simulink model "intento2"  (R2017b)
settings: Solver=VariableStepAuto  StartTime=0.0  StopTime=10.0  RelTol=1e-3
values from neighbouring files (symbols this model uses):
  kd = eval(S.kd)    [Lab4.m]    (also in Lab4Final.m; Lab4intento2.m; Lab4intento3.m)
  ki = eval(S.ki)    [Lab4.m]    (also in Lab4Final.m; Lab4intento2.m; Lab4intento3.m)
  ki2 = eval(S.ki2)    [Lab4Final.m]    (also in Lab4intento2.m)
  ki3 = eval(S.ki3)    [Lab4intento2.m]
  kp = eval(S.kp)    [Lab4.m]    (also in Lab4Final.m; Lab4intento2.m; Lab4intento3.m)
settings Model: Creator=Cx001la  LastModifiedBy=Cx001la

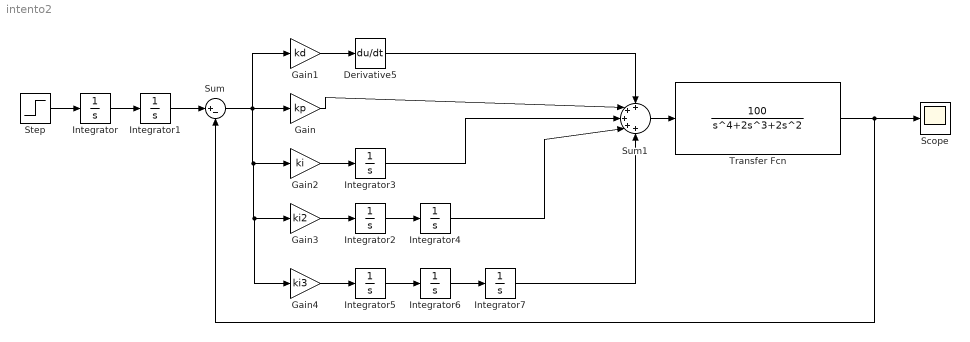
== system intento2 ==
  Derivative5 : Derivative
  Gain : Gain  Gain=kp
  Gain1 : Gain  Gain=kd
  Gain2 : Gain  Gain=ki
  Gain3 : Gain  Gain=ki2
  Gain4 : Gain  Gain=ki3
  Integrator{,1..7} (8 alike) : Integrator
  Scope : Scope
  Step : Step  Time=0  SampleTime=0
  Sum : Sum  Inputs=|+-
  Sum1 : Sum  Inputs=+++++
  Transfer Fcn : TransferFcn  Numerator=[100]  Denominator=[1 2 2 0 0]
  wires:
  Transfer Fcn/1 -> Scope/1, Sum/2
  Sum1/1 -> Transfer Fcn/1
  Integrator1/1 -> Sum/1
  Step/1 -> Integrator/1
  Sum/1 -> Gain1/1, Gain4/1, Gain3/1, Gain2/1, Gain/1
  Integrator/1 -> Integrator1/1
  Gain/1 -> Sum1/2
  Gain1/1 -> Derivative5/1
  Derivative5/1 -> Sum1/1
  Gain2/1 -> Integrator3/1
  Gain3/1 -> Integrator2/1
  Integrator2/1 -> Integrator4/1
  Gain4/1 -> Integrator5/1
  Integrator5/1 -> Integrator6/1
  Integrator6/1 -> Integrator7/1
  Integrator7/1 -> Sum1/5
  Integrator4/1 -> Sum1/4
  Integrator3/1 -> Sum1/3
